simulink model "Sistema"  (R2013a)
settings: Solver=FixedStepDiscrete  StartTime=0.0  StopTime=10.0  FixedStep=30E-3  RelTol=1e-3
libraries: dspnetwork x3
settings Model: Creator=vmaraccini-personal  LastModifiedBy=vmaraccini-personal

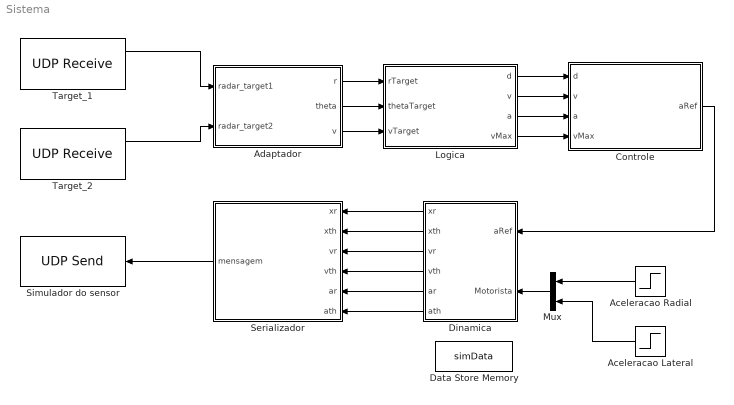
== system Sistema ==
  Aceleracao Lateral : Step  Time=2  After=-3  SampleTime=0
  Aceleracao Radial : Step  Time=2  After=-3  SampleTime=0
  Adaptador : MATLAB Function  TreatAsAtomicUnit=on
  Controle : MATLAB Function  TreatAsAtomicUnit=on
  Data Store Memory : DataStoreMemory  DataStoreName=simData  ReadBeforeWriteMsg=warning  WriteAfterWriteMsg=warning  WriteAfterReadMsg=warning  InitialValue=[0 0 0 0 0 0]  OutDataTypeStr=double
  Dinamica : MATLAB Function  TreatAsAtomicUnit=on
  Logica : MATLAB Function  TreatAsAtomicUnit=on
  Mux : Mux  Inputs=2
  Serializador : MATLAB Function  TreatAsAtomicUnit=on
  Simulador do sensor : dspnetwork/UDP Send  remoteURL='127.0.0.1'  remotePort=25000  localURL='0.0.0.0'  localPortSource=Automatically determine  localPort=-1  sampletime=-1  separateLengthPort=0
  Target_1 : dspnetwork/UDP Receive  localURL='0.0.0.0'  localPort=25000  remoteURL='0.0.0.0'  remotePort=-1  recvBufferSize=8192  dims=3000  signalDatatype=uint8  isVarSize=off  showBlockingTime=off  blockingTime=0  sampletime=0.03
  Target_2 : dspnetwork/UDP Receive  localURL='0.0.0.0'  localPort=25001  remoteURL='0.0.0.0'  remotePort=-1  recvBufferSize=8192  dims=3000  signalDatatype=uint8  isVarSize=off  showBlockingTime=off  blockingTime=0  sampletime=0.03
  wires:
  Serializador/1(mensagem) -> Simulador do sensor/1
  Target_1/1 -> Adaptador/1(radar_target1)
  Target_2/1 -> Adaptador/2(radar_target2)
  Adaptador/1(r) -> Logica/1(rTarget)
  Adaptador/2(theta) -> Logica/2(thetaTarget)
  Adaptador/3(v) -> Logica/3(vTarget)
  Logica/1(d) -> Controle/1(d)
  Logica/4(vMax) -> Controle/4(vMax)
  Logica/3(a) -> Controle/3(a)
  Logica/2(v) -> Controle/2(v)
  Controle/1(aRef) -> Dinamica/1(aRef)
  Dinamica/1(xr) -> Serializador/1(xr)
  Dinamica/2(xth) -> Serializador/2(xth)
  Dinamica/3(vr) -> Serializador/3(vr)
  Dinamica/4(vth) -> Serializador/4(vth)
  Dinamica/5(ar) -> Serializador/5(ar)
  Dinamica/6(ath) -> Serializador/6(ath)
  Mux/1 -> Dinamica/2(Motorista)
  Aceleracao Radial/1 -> Mux/1
  Aceleracao Lateral/1 -> Mux/2

== matlab function Sistema/Adaptador ==
  data: radar_target1 input; r output; radar_target2 input; theta output; v output
function [ r, theta, v ] = Adaptador( radar_target1, radar_target2 )
r = [0 0 0];
theta = [0 0 0];
v = [0 0 0];
% [r, theta, v] = RadarAdapter(parse_json(radar_target1), parse_json(radar_target2));
end

== matlab function Sistema/Serializador ==
  data: xr input; mensagem output; xth input; vr input; vth input; ar input; ath input
function mensagem  = Serializa(xr, xth, vr, vth, ar, ath)
%SERIALIZA: Adapta os dados de simulacao para serem transmitidos
mensagem = uint8('0');
end

== matlab function Sistema/Logica ==
  data: rTarget input; d output; thetaTarget input; vTarget input; v output; a output; vMax output
function [d, v, a, vMax] = Logica(rTarget, thetaTarget, vTarget)
%#Logica de interpretacao

% [d, v, a, vMax] = intepreta(rTarget, thetaTarget, vTarget);
d = 0;
v = 0;
a = 0;
vMax = 0;

end

== matlab function Sistema/Controle ==
  data: d input; v input; a input; vMax input; aRef output
function aRef  = Controle(d, v, a, vMax)
%#Logica de interpretacao

aRef = 0;

end

== matlab function Sistema/Dinamica ==
  data: aRef input; xr output; xth output; vr output; vth output; Motorista input; ar output; ath output; simData data_store_memory
function [xr, xth, vr, vth, ar, ath] = Dinamica(aRef, Motorista)
%DINAMICA: Calcula a posicao futura dos veiculos

global simData;
xrD = simData(1);
xthD = simData(2);
vrD = simData(3);
vthD = simData(4);
arD = simData(5);
athD = simData(6);

step = 30E-3

ar = arD - aRef;
ath = athD;

vr = vrD + step * ar;
vth = vthD + step * athD;

xr = xrD + step * vr;
xth = xthD + step * vth;

%Primeiro carro eh o carro sendo seguido
ar(1) = ar(1) + Motorista(1);
ath(1) = ath(1) + Motorista(2);

%Atualizar valores globais
simData = [xrD, xthD, vrD, vthD, arD, athD]';

end
